simulink subsystem "PvtSubSys_PLAN_ALC"  (R2020b)
settings: Solver=VariableStepAuto  StartTime=0.0  StopTime=10.0  RelTol=1e-3
undefined symbols (not defined in the file or in its folder): P_Global_WheelBase_m, P_Global_WheelTrack_m, P_PLAN_ALC_DPCConfirmTimeHMI, P_PLAN_ALC_DPCExtraMultiFrameConfirmCntDrv, P_PLAN_ALC_DPCExtraMultiFrameConfirmCntNoh, P_PLAN_ALC_DPCExtraMultiFrameConfirmCntOverTk, P_PLAN_ALC_DPCthresholdLcDrvLv1, P_PLAN_ALC_DPCthresholdLcDrvLv2, P_PLAN_ALC_DPCthresholdLcDrvLv3, P_PLAN_ALC_DynamicDPCthreshold, P_PLAN_ALC_FWheelPreTime, P_PLAN_ALC_LcCancelDPCThreshold, P_PLAN_ALC_LcCancelLaneChangeReqDspTimeCnt, P_PLAN_ALC_LcCancelRoadWidthOffset, P_PLAN_ALC_LcCancelRoadWidthOffsetForDPC, P_PLAN_ALC_LcCurvatureInhibitionValueBrkPoints, P_PLAN_ALC_LcCurvatureInhibitionValueTable, P_PLAN_ALC_LcDelayCntSetNoh, P_PLAN_ALC_LcDelayCntSetOverTk, P_PLAN_ALC_LCDeltaTmeGap, P_PLAN_ALC_LcDrv_DyDiffThreshold, P_PLAN_ALC_LcDrvHMILineValidFtime, P_PLAN_ALC_LcEnterLane_factor, P_PLAN_ALC_LcFinishDyDiffBrkPoint, P_PLAN_ALC_LcFinishDyDiffRwFactorForAP, P_PLAN_ALC_LcFinishDyDiffRwFactorForHMI, P_PLAN_ALC_LcFinishDyDiffTableValue, P_PLAN_ALC_LciDrvExistDefaultDisp, P_PLAN_ALC_LciOverTkDeltaSpdLv1, P_PLAN_ALC_LciOverTkDeltaSpdLv2, P_PLAN_ALC_LciOverTkDeltaSpdLv3, P_PLAN_ALC_LcOverTkDPCthreshold, P_PLAN_ALC_LcOverTkRearVehTTClimit, P_PLAN_ALC_NOHLcSwt, P_PLAN_ALC_NOHTurnSts, P_PLAN_ALC_OverTkCutOutDyRWFactor, P_PLAN_ALC_OveTkrSupDist, P_PLAN_ALC_PreCurvatureFactor, P_PLAN_ALC_PreCurvaturePreTime, P_PLAN_ALC_TurnLmpType, P_PLAN_ALC_vMinPreLC_Drv, P_PLAN_ALC_vMinPreLC_Noh, P_PLAN_ALC_vMinPreLC_OverTk, P_PLAN_LcCancelTestEnable, PLAN_ALC_DangerObjIndex, PLAN_ALC_LcCancelReason, PLAN_ALC_LcDecsLe, PLAN_ALC_LcDecsRi, PLAN_ALC_LcFeReason, PLAN_ALC_LcReason, PLAN_ALC_sts, PLAN_ALC_stsReason, PLAN_ALC_TurnLightReq
libraries: simulink x198, TrueDurationTime x21, RisingEdgeTimer x2, JumpDetectionUint x1
(part 4 of 4)

== system PvtSubSys_PLAN_ALC/PLAN_IPHMI/Subsystem1 ==
  note: 0x1:need to lanechange but Conds not Satisfied
      | 0x2: ready to lanechange
  note: 该信号表示存在换道指示但不满足部分条件
  In1 : Inport
  LineValid : Inport  Port=2
  DPC : Inport  Port=3
  DPC_OnComing : Inport  Port=4
  LciDrvRi : Inport  Port=5
  AND : Logic  Commented=on  Inputs=4  AllPortsSameDT=off  OutDataTypeStr=boolean
  AND1 : Logic  Commented=on  AllPortsSameDT=off  OutDataTypeStr=boolean
  AND4 : Logic  AllPortsSameDT=off  OutDataTypeStr=boolean
  Bus Selector1 : BusSelector  Commented=on  OutputSignals=PLAN_ALC_LcDrvLe_IPVehSpd,PLAN_ALC_LcDrvLe_NoOnComing,PLAN_ALC_LcDrvLe_DPC,PLAN_ALC_LcDrvLe_LineValid,PLAN_ALC_LcDrvLe_LciDrv
  Chart1 : Stateflow chart  Commented=on  TreatAsAtomicUnit=on
  Chart2 : Stateflow chart  Commented=on  TreatAsAtomicUnit=on
  Compare To Constant : simulink/Logic and Bit Operations/Compare To Constant  Commented=on  relop=<=  const=P_PLAN_ALC_LcDrvHMILineValidFtime  OutDataTypeStr=boolean
  Compare To Constant1 : simulink/Logic and Bit Operations/Compare To Constant  relop=>  const=P_PLAN_ALC_LcDrvHMILineValidFtime  OutDataTypeStr=boolean
  Compare To Constant2 : simulink/Logic and Bit Operations/Compare To Constant  relop=>  const=P_PLAN_ALC_DynamicDPCthreshold  OutDataTypeStr=boolean
  Compare To Constant3 : simulink/Logic and Bit Operations/Compare To Constant  Commented=on  relop=<  const=P_PLAN_ALC_DynamicDPCthreshold  OutDataTypeStr=boolean
  Compare To Constant4 : simulink/Logic and Bit Operations/Compare To Constant  Commented=on  relop=>  const=P_PLAN_ALC_DPCConfirmTimeHMI  OutDataTypeStr=boolean
  Compare To Constant5 : simulink/Logic and Bit Operations/Compare To Constant  relop=>  const=P_PLAN_ALC_LcDrvHMILineValidFtime  OutDataTypeStr=boolean
  Constant7 : Constant  OutDataTypeStr=uint8
  Constant8 : Constant  Value=P_PLAN_ALC_LciDrvExistDefaultDisp  OutDataTypeStr=uint8
  Constant9 : Constant  Value=0  OutDataTypeStr=uint8
  NOT : Logic  Commented=on  Operator=NOT  IconShape=distinctive  AllPortsSameDT=off  OutDataTypeStr=boolean
  NOT1 : Logic  Operator=NOT  IconShape=distinctive  AllPortsSameDT=off  OutDataTypeStr=boolean
  NOT2 : Logic  Operator=NOT  IconShape=distinctive  AllPortsSameDT=off  OutDataTypeStr=boolean
  OR : Logic  Commented=on  Operator=OR  AllPortsSameDT=off  OutDataTypeStr=boolean
  OR1 : Logic  Commented=on  Operator=OR  AllPortsSameDT=off  OutDataTypeStr=boolean
  OR2 : Logic  Operator=OR  Inputs=4  AllPortsSameDT=off  OutDataTypeStr=boolean
  OR4 : Logic  AllPortsSameDT=off  OutDataTypeStr=boolean
  Switch : Switch  Criteria=u2 ~= 0
  Switch1 : Switch  Criteria=u2 ~= 0
  Terminator : Terminator  Commented=on
  TrueDurationTime1 : TrueDurationTime/TrueDurationTime  TCycle=0.02
  TrueDurationTime2 : TrueDurationTime/TrueDurationTime  Commented=on  TCycle=0.02
  TrueDurationTime3 : TrueDurationTime/TrueDurationTime  Commented=on  TCycle=0.02
  TrueDurationTime4 : TrueDurationTime/TrueDurationTime  TCycle=0.02
  LcDrvSatisfiedStsRi : Outport
  wires:
  Compare To Constant5/1 -> OR2/3
  TrueDurationTime4/1 -> Compare To Constant5/1
  NOT1/1 -> TrueDurationTime4/1
  In1/1 -> NOT1/1
  TrueDurationTime2/1 -> Compare To Constant4/1
  Compare To Constant3/1 -> TrueDurationTime2/1
  Chart2/1(LcSts) -> Terminator/1
  OR/1 -> AND/3
  OR1/1 -> AND/4
  NOT/1 -> AND1/2, TrueDurationTime3/1
  TrueDurationTime3/1 -> Compare To Constant/1
  AND1/1 -> OR/2, OR1/2
  AND/1 -> Chart2/1(LcConds)
  Compare To Constant/1 -> AND1/1
  DPC_OnComing/1 -> OR2/4
  Constant9/1 -> Switch1/3
  Bus Selector1/3 -> OR/1  "<PLAN_ALC_LcDrvLe_DPC>"
  AND4/1 -> Switch/2
  Bus Selector1/4 -> NOT/1, OR1/1  "<PLAN_ALC_LcDrvLe_LineValid>"
  Constant8/1 -> Switch1/1
  OR2/1 -> AND4/1  "LcNotSatisfied"
  Switch1/1 -> Switch/3
  NOT2/1 -> TrueDurationTime1/1
  TrueDurationTime1/1 -> Compare To Constant1/1
  Compare To Constant1/1 -> OR2/2
  Bus Selector1/1 -> AND/1  "<PLAN_ALC_LcDrvLe_IPVehSpd>"
  Constant7/1 -> Switch/1
  Bus Selector1/2 -> AND/2  "<PLAN_ALC_LcDrvLe_NoOnComing>"
  Compare To Constant2/1 -> OR4/1
  LineValid/1 -> OR4/2, NOT2/1
  Switch/1 -> LcDrvSatisfiedStsRi/1  "LcDrvSatisfiedStsRi"
  LciDrvRi/1 -> Switch1/2, AND4/2
  Bus Selector1/5 -> Chart2/2(LcReq)  "<PLAN_ALC_LcDrvLe_LciDrv>"
  DPC/1 -> Compare To Constant2/1
  Compare To Constant4/1 -> Chart1/1(on)
  OR4/1 -> OR2/1

== system PvtSubSys_PLAN_ALC/PLAN_IPHMI/Subsystem2 ==
  note: 0x1:need to lanechange but Conds not Satisfied
      | 0x2: ready to lanechange
  note: 该信号表示存在换道指示但不满足部分条件
  LineValid : Inport
  DPC : Inport  Port=2
  LciDrvLe : Inport  Port=3
  AND : Logic  Commented=on  Inputs=4  AllPortsSameDT=off  OutDataTypeStr=boolean
  AND1 : Logic  Commented=on  AllPortsSameDT=off  OutDataTypeStr=boolean
  AND4 : Logic  AllPortsSameDT=off  OutDataTypeStr=boolean
  Bus Selector1 : BusSelector  Commented=on  OutputSignals=PLAN_ALC_LcDrvLe_IPVehSpd,PLAN_ALC_LcDrvLe_NoOnComing,PLAN_ALC_LcDrvLe_DPC,PLAN_ALC_LcDrvLe_LineValid,PLAN_ALC_LcDrvLe_LciDrv
  Chart1 : Stateflow chart  Commented=on  TreatAsAtomicUnit=on
  Chart2 : Stateflow chart  Commented=on  TreatAsAtomicUnit=on
  Compare To Constant : simulink/Logic and Bit Operations/Compare To Constant  Commented=on  relop=<=  const=P_PLAN_ALC_LcDrvHMILineValidFtime  OutDataTypeStr=boolean
  Compare To Constant2 : simulink/Logic and Bit Operations/Compare To Constant  relop=>  const=P_PLAN_ALC_DynamicDPCthreshold  OutDataTypeStr=boolean
  Compare To Constant3 : simulink/Logic and Bit Operations/Compare To Constant  Commented=on  relop=<  const=P_PLAN_ALC_DynamicDPCthreshold  OutDataTypeStr=boolean
  Compare To Constant4 : simulink/Logic and Bit Operations/Compare To Constant  Commented=on  relop=>  const=P_PLAN_ALC_DPCConfirmTimeHMI  OutDataTypeStr=boolean
  Constant7 : Constant  OutDataTypeStr=uint8
  Constant8 : Constant  Value=P_PLAN_ALC_LciDrvExistDefaultDisp  OutDataTypeStr=uint8
  Constant9 : Constant  Value=0  OutDataTypeStr=uint8
  NOT : Logic  Commented=on  Operator=NOT  IconShape=distinctive  AllPortsSameDT=off  OutDataTypeStr=boolean
  OR : Logic  Commented=on  Operator=OR  AllPortsSameDT=off  OutDataTypeStr=boolean
  OR1 : Logic  Commented=on  Operator=OR  AllPortsSameDT=off  OutDataTypeStr=boolean
  OR4 : Logic  AllPortsSameDT=off  OutDataTypeStr=boolean
  Switch : Switch  Criteria=u2 ~= 0
  Switch1 : Switch  Criteria=u2 ~= 0
  Terminator : Terminator  Commented=on
  TrueDurationTime2 : TrueDurationTime/TrueDurationTime  Commented=on  TCycle=0.02
  TrueDurationTime3 : TrueDurationTime/TrueDurationTime  Commented=on  TCycle=0.02
  LcNohSatisfiedStsLe : Outport
  wires:
  TrueDurationTime2/1 -> Compare To Constant4/1
  Compare To Constant3/1 -> TrueDurationTime2/1
  Chart2/1(LcSts) -> Terminator/1
  OR/1 -> AND/3
  OR1/1 -> AND/4
  NOT/1 -> AND1/2, TrueDurationTime3/1
  TrueDurationTime3/1 -> Compare To Constant/1
  AND1/1 -> OR/2, OR1/2
  AND/1 -> Chart2/1(LcConds)
  Compare To Constant/1 -> AND1/1
  Constant9/1 -> Switch1/3
  Bus Selector1/3 -> OR/1  "<PLAN_ALC_LcDrvLe_DPC>"
  AND4/1 -> Switch/2
  Bus Selector1/4 -> NOT/1, OR1/1  "<PLAN_ALC_LcDrvLe_LineValid>"
  Constant8/1 -> Switch1/1
  OR4/1 -> AND4/1  "LcNotSatisfied"
  Switch1/1 -> Switch/3
  Bus Selector1/1 -> AND/1  "<PLAN_ALC_LcDrvLe_IPVehSpd>"
  Constant7/1 -> Switch/1
  Bus Selector1/2 -> AND/2  "<PLAN_ALC_LcDrvLe_NoOnComing>"
  Compare To Constant2/1 -> OR4/1
  LineValid/1 -> OR4/2
  Switch/1 -> LcNohSatisfiedStsLe/1  "LcNohSatisfiedStsLe"
  LciDrvLe/1 -> Switch1/2, AND4/2
  Bus Selector1/5 -> Chart2/2(LcReq)  "<PLAN_ALC_LcDrvLe_LciDrv>"
  DPC/1 -> Compare To Constant2/1
  Compare To Constant4/1 -> Chart1/1(on)

== system PvtSubSys_PLAN_ALC/PLAN_IPHMI/Subsystem3 ==
  note: 0x1:need to lanechange but Conds not Satisfied
      | 0x2: ready to lanechange
  note: 该信号表示存在换道指示但不满足部分条件
  LineValid : Inport
  DPC : Inport  Port=2
  LciDrvRi : Inport  Port=3
  AND : Logic  Commented=on  Inputs=4  AllPortsSameDT=off  OutDataTypeStr=boolean
  AND1 : Logic  Commented=on  AllPortsSameDT=off  OutDataTypeStr=boolean
  AND4 : Logic  AllPortsSameDT=off  OutDataTypeStr=boolean
  Bus Selector1 : BusSelector  Commented=on  OutputSignals=PLAN_ALC_LcDrvLe_IPVehSpd,PLAN_ALC_LcDrvLe_NoOnComing,PLAN_ALC_LcDrvLe_DPC,PLAN_ALC_LcDrvLe_LineValid,PLAN_ALC_LcDrvLe_LciDrv
  Chart1 : Stateflow chart  Commented=on  TreatAsAtomicUnit=on
  Chart2 : Stateflow chart  Commented=on  TreatAsAtomicUnit=on
  Compare To Constant : simulink/Logic and Bit Operations/Compare To Constant  Commented=on  relop=<=  const=P_PLAN_ALC_LcDrvHMILineValidFtime  OutDataTypeStr=boolean
  Compare To Constant2 : simulink/Logic and Bit Operations/Compare To Constant  relop=>  const=P_PLAN_ALC_DynamicDPCthreshold  OutDataTypeStr=boolean
  Compare To Constant3 : simulink/Logic and Bit Operations/Compare To Constant  Commented=on  relop=<  const=P_PLAN_ALC_DynamicDPCthreshold  OutDataTypeStr=boolean
  Compare To Constant4 : simulink/Logic and Bit Operations/Compare To Constant  Commented=on  relop=>  const=P_PLAN_ALC_DPCConfirmTimeHMI  OutDataTypeStr=boolean
  Constant7 : Constant  OutDataTypeStr=uint8
  Constant8 : Constant  Value=P_PLAN_ALC_LciDrvExistDefaultDisp  OutDataTypeStr=uint8
  Constant9 : Constant  Value=0  OutDataTypeStr=uint8
  NOT : Logic  Commented=on  Operator=NOT  IconShape=distinctive  AllPortsSameDT=off  OutDataTypeStr=boolean
  OR : Logic  Commented=on  Operator=OR  AllPortsSameDT=off  OutDataTypeStr=boolean
  OR1 : Logic  Commented=on  Operator=OR  AllPortsSameDT=off  OutDataTypeStr=boolean
  OR4 : Logic  AllPortsSameDT=off  OutDataTypeStr=boolean
  Switch : Switch  Criteria=u2 ~= 0
  Switch1 : Switch  Criteria=u2 ~= 0
  Terminator : Terminator  Commented=on
  TrueDurationTime2 : TrueDurationTime/TrueDurationTime  Commented=on  TCycle=0.02
  TrueDurationTime3 : TrueDurationTime/TrueDurationTime  Commented=on  TCycle=0.02
  LcNohSatisfiedStsRi : Outport
  wires:
  TrueDurationTime2/1 -> Compare To Constant4/1
  Compare To Constant3/1 -> TrueDurationTime2/1
  Chart2/1(LcSts) -> Terminator/1
  OR/1 -> AND/3
  OR1/1 -> AND/4
  NOT/1 -> AND1/2, TrueDurationTime3/1
  TrueDurationTime3/1 -> Compare To Constant/1
  AND1/1 -> OR/2, OR1/2
  AND/1 -> Chart2/1(LcConds)
  Compare To Constant/1 -> AND1/1
  Constant9/1 -> Switch1/3
  Bus Selector1/3 -> OR/1  "<PLAN_ALC_LcDrvLe_DPC>"
  AND4/1 -> Switch/2
  Bus Selector1/4 -> NOT/1, OR1/1  "<PLAN_ALC_LcDrvLe_LineValid>"
  Constant8/1 -> Switch1/1
  OR4/1 -> AND4/1  "LcNotSatisfied"
  Switch1/1 -> Switch/3
  Bus Selector1/1 -> AND/1  "<PLAN_ALC_LcDrvLe_IPVehSpd>"
  Constant7/1 -> Switch/1
  Bus Selector1/2 -> AND/2  "<PLAN_ALC_LcDrvLe_NoOnComing>"
  Compare To Constant2/1 -> OR4/1
  LineValid/1 -> OR4/2
  Switch/1 -> LcNohSatisfiedStsRi/1  "LcNohSatisfiedStsRi"
  LciDrvRi/1 -> Switch1/2, AND4/2
  Bus Selector1/5 -> Chart2/2(LcReq)  "<PLAN_ALC_LcDrvLe_LciDrv>"
  DPC/1 -> Compare To Constant2/1
  Compare To Constant4/1 -> Chart1/1(on)

== system PvtSubSys_PLAN_ALC/PLAN_IPHMI/Subsystem4 ==
  note: 该信号表示存在换道指示但不满足部分条件
  note: 0x1:need to lanechange but Conds not Satisfied
      | 0x2: ready to lanechange
  LineValid : Inport
  DPC : Inport  Port=2
  LciDrvRi : Inport  Port=3
  AND : Logic  Commented=on  Inputs=4  AllPortsSameDT=off  OutDataTypeStr=boolean
  AND1 : Logic  Commented=on  AllPortsSameDT=off  OutDataTypeStr=boolean
  AND4 : Logic  AllPortsSameDT=off  OutDataTypeStr=boolean
  Bus Selector1 : BusSelector  Commented=on  OutputSignals=PLAN_ALC_LcDrvLe_IPVehSpd,PLAN_ALC_LcDrvLe_NoOnComing,PLAN_ALC_LcDrvLe_DPC,PLAN_ALC_LcDrvLe_LineValid,PLAN_ALC_LcDrvLe_LciDrv
  Chart1 : Stateflow chart  Commented=on  TreatAsAtomicUnit=on
  Chart2 : Stateflow chart  Commented=on  TreatAsAtomicUnit=on
  Compare To Constant : simulink/Logic and Bit Operations/Compare To Constant  Commented=on  relop=<=  const=P_PLAN_ALC_LcDrvHMILineValidFtime  OutDataTypeStr=boolean
  Compare To Constant1 : simulink/Logic and Bit Operations/Compare To Constant  relop=>  const=P_PLAN_ALC_LcDrvHMILineValidFtime  OutDataTypeStr=boolean
  Compare To Constant2 : simulink/Logic and Bit Operations/Compare To Constant  relop=>  const=P_PLAN_ALC_DynamicDPCthreshold  OutDataTypeStr=boolean
  Compare To Constant3 : simulink/Logic and Bit Operations/Compare To Constant  Commented=on  relop=<  const=P_PLAN_ALC_DynamicDPCthreshold  OutDataTypeStr=boolean
  Compare To Constant4 : simulink/Logic and Bit Operations/Compare To Constant  Commented=on  relop=>  const=P_PLAN_ALC_DPCConfirmTimeHMI  OutDataTypeStr=boolean
  Constant7 : Constant  OutDataTypeStr=uint8
  Constant8 : Constant  Value=P_PLAN_ALC_LciDrvExistDefaultDisp  OutDataTypeStr=uint8
  Constant9 : Constant  Value=0  OutDataTypeStr=uint8
  Ground : Ground
  NOT : Logic  Commented=on  Operator=NOT  IconShape=distinctive  AllPortsSameDT=off  OutDataTypeStr=boolean
  NOT2 : Logic  Operator=NOT  IconShape=distinctive  AllPortsSameDT=off  OutDataTypeStr=boolean
  OR : Logic  Commented=on  Operator=OR  AllPortsSameDT=off  OutDataTypeStr=boolean
  OR1 : Logic  Commented=on  Operator=OR  AllPortsSameDT=off  OutDataTypeStr=boolean
  OR2 : Logic  Operator=OR  Inputs=3  AllPortsSameDT=off  OutDataTypeStr=boolean
  OR4 : Logic  AllPortsSameDT=off  OutDataTypeStr=boolean
  Switch : Switch  Criteria=u2 ~= 0
  Switch1 : Switch  Criteria=u2 ~= 0
  Terminator : Terminator  Commented=on
  TrueDurationTime1 : TrueDurationTime/TrueDurationTime  TCycle=0.02
  TrueDurationTime2 : TrueDurationTime/TrueDurationTime  Commented=on  TCycle=0.02
  TrueDurationTime3 : TrueDurationTime/TrueDurationTime  Commented=on  TCycle=0.02
  LcMrcSatisfiedStsRi : Outport
  wires:
  OR4/1 -> OR2/1
  Compare To Constant4/1 -> Chart1/1(on)
  DPC/1 -> Compare To Constant2/1
  Bus Selector1/5 -> Chart2/2(LcReq)  "<PLAN_ALC_LcDrvLe_LciDrv>"
  LciDrvRi/1 -> AND4/2, Switch1/2
  Switch/1 -> LcMrcSatisfiedStsRi/1  "LcNohSatisfiedStsRi"
  LineValid/1 -> NOT2/1, OR4/2
  Compare To Constant2/1 -> OR4/1
  Bus Selector1/2 -> AND/2  "<PLAN_ALC_LcDrvLe_NoOnComing>"
  Constant7/1 -> Switch/1
  Bus Selector1/1 -> AND/1  "<PLAN_ALC_LcDrvLe_IPVehSpd>"
  Compare To Constant1/1 -> OR2/2
  TrueDurationTime1/1 -> Compare To Constant1/1
  NOT2/1 -> TrueDurationTime1/1
  Switch1/1 -> Switch/3
  OR2/1 -> AND4/1  "LcNotSatisfied"
  Constant8/1 -> Switch1/1
  Bus Selector1/4 -> OR1/1, NOT/1  "<PLAN_ALC_LcDrvLe_LineValid>"
  AND4/1 -> Switch/2
  Bus Selector1/3 -> OR/1  "<PLAN_ALC_LcDrvLe_DPC>"
  Constant9/1 -> Switch1/3
  Compare To Constant/1 -> AND1/1
  AND/1 -> Chart2/1(LcConds)
  AND1/1 -> OR1/2, OR/2
  TrueDurationTime3/1 -> Compare To Constant/1
  NOT/1 -> TrueDurationTime3/1, AND1/2
  OR1/1 -> AND/4
  OR/1 -> AND/3
  Chart2/1(LcSts) -> Terminator/1
  Compare To Constant3/1 -> TrueDurationTime2/1
  TrueDurationTime2/1 -> Compare To Constant4/1
  Ground/1 -> OR2/3

== system PvtSubSys_PLAN_ALC/LcCancelFinishCalc1/Subsystem3/LPF ==
  signal : Inport
  Constant1 : Constant  Value=0.1
  MATLAB Function2 : MATLAB Function  TreatAsAtomicUnit=on
  Unit Delay2 : UnitDelay  SampleTime=-1  HasFrameUpgradeWarning=on
  result : Outport
  wires:
  MATLAB Function2/1(result) -> result/1, Unit Delay2/1
  Unit Delay2/1 -> MATLAB Function2/3(resultK1)
  Constant1/1 -> MATLAB Function2/1(Alpha)
  signal/1 -> MATLAB Function2/2(signal)

== system PvtSubSys_PLAN_ALC/LcCancelFinishCalc1/Subsystem3/Simulink Function ==
  note: 预测车体上的点或者固连在车体上的点的位置
  f : TriggerPort  TriggerType=function-call  IsSimulinkFunction=on  FunctionName=PointPre  FunctionVisibility=scoped  VariantControl=(inherit)
  Bus Selector : BusSelector  OutputSignals=mPrePointX,mPrePointY
  Bus Creator : BusCreator  Inputs=2
  Bus Creator1 : BusCreator  Inputs=2
  If : If  IfExpression=u1 == 0
  Merge : Merge
  Subsystem : Subsystem
  Subsystem1 : Subsystem
  u : ArgIn  DisableCoverage=on  OutDataTypeStr=single  ArgumentName=mPointX
  u1 : ArgIn  DisableCoverage=on  Port=2  OutDataTypeStr=single  ArgumentName=mPointY
  u2 : ArgIn  DisableCoverage=on  Port=3  OutDataTypeStr=single  ArgumentName=kapTraj
  u3 : ArgIn  DisableCoverage=on  Port=4  OutDataTypeStr=single  ArgumentName=mpsTrajSpd
  u4 : ArgIn  DisableCoverage=on  Port=5  OutDataTypeStr=single  ArgumentName=sPreTime
  y : ArgOut  DisableCoverage=on  OutDataTypeStr=single  ArgumentName=mPrePointX
  y1 : ArgOut  DisableCoverage=on  Port=2  OutDataTypeStr=single  ArgumentName=mPrePointY
  wires:
  Subsystem/1(mPrePointX) -> Bus Creator/1
  If/1 -> Subsystem1/Action
  Subsystem1/2(mPrePointY) -> Bus Creator1/2
  Subsystem1/1(mPrePointX) -> Bus Creator1/1
  u3/1 -> Subsystem1/1(mpsTrajSpd), Subsystem/2(mpsTrajSpd)
  Bus Creator/1 -> Merge/1
  Bus Selector/2 -> y1/1  "<mPrePointY>"
  Subsystem/2(mPrePointY) -> Bus Creator/2
  Merge/1 -> Bus Selector/1
  u/1 -> Subsystem1/3(mPointX), Subsystem/4(mPointX)
  u2/1 -> If/1, Subsystem/1(kapTraj)
  If/2 -> Subsystem/Action
  u4/1 -> Subsystem1/2(sPreTime), Subsystem/3(sPreTime)
  u1/1 -> Subsystem1/4(mPointY), Subsystem/5(mPointY)
  Bus Selector/1 -> y/1  "<mPrePointX>"
  Bus Creator1/1 -> Merge/2

== system PvtSubSys_PLAN_ALC/LcCancelFinishCalc1/Subsystem3/Simulink Function1 ==
  FrenetCS : TriggerPort  TriggerType=function-call  IsSimulinkFunction=on  FunctionName=FrenetCS  FunctionVisibility=scoped  VariantControl=(inherit)
  Add : Sum  Inputs=+++
  Add1 : Sum
  Add2 : Sum
  Constant : Constant  OutDataTypeStr=Inherit: Inherit via back propagation
  Divide : Product  Inputs=*/
  Gain : Gain  Gain=2
  Math Function : Math  Operator=square  SaturateOnIntegerOverflow=on
  Math Function1 : Math  Operator=square  SaturateOnIntegerOverflow=on
  Product : Product
  Product1 : Product
  Product2 : Product
  Sqrt : Sqrt  SaturateOnIntegerOverflow=on
  Subtract1 : Sum  Inputs=+-
  u : ArgIn  DisableCoverage=on  OutDataTypeStr=single  ArgumentName=LaneC0
  u1 : ArgIn  DisableCoverage=on  Port=2  OutDataTypeStr=single  ArgumentName=LaneC1
  u2 : ArgIn  DisableCoverage=on  Port=3  OutDataTypeStr=single  ArgumentName=LaneC2
  u4 : ArgIn  DisableCoverage=on  Port=4  OutDataTypeStr=single  ArgumentName=PointX
  u5 : ArgIn  DisableCoverage=on  Port=5  OutDataTypeStr=single  ArgumentName=PointY
  y1 : ArgOut  DisableCoverage=on  OutDataTypeStr=single  ArgumentName=PointFrenetD
  wires:
  u1/1 -> Add1/1, Product/2
  u4/1 -> Product/1, Math Function/1, Product2/2
  u2/1 -> Product1/2, Product2/1
  Math Function/1 -> Product1/1
  Product/1 -> Add/1
  Product1/1 -> Add/2
  u/1 -> Add/3
  Product2/1 -> Gain/1
  Gain/1 -> Add1/2
  Add1/1 -> Math Function1/1
  Math Function1/1 -> Add2/1
  Constant/1 -> Add2/2
  Add2/1 -> Sqrt/1
  Add/1 -> Subtract1/2
  Sqrt/1 -> Divide/2
  u5/1 -> Subtract1/1
  Divide/1 -> y1/1
  Subtract1/1 -> Divide/1

== system PvtSubSys_PLAN_ALC/LcOverTk/Subsystem5/Counter1 ==
  Trigger : Inport
  Constant3 : Constant  OutDataTypeStr=uint16
  Constant4 : Constant  Value=0  OutDataTypeStr=uint16
  Saturation1 : Saturate  UpperLimit=65000  LowerLimit=0
  Sum : Sum  Inputs=++|
  Switch : Switch  Criteria=u2 ~= 0
  Switch1 : Switch  Criteria=u2 ~= 0
  Unit Delay : UnitDelay  SampleTime=-1  HasFrameUpgradeWarning=on
  Cnt : Outport
  wires:
  Constant4/1 -> Switch/3, Switch1/3
  Constant3/1 -> Switch/1
  Switch1/1 -> Saturation1/1
  Switch/1 -> Sum/2
  Unit Delay/1 -> Sum/1
  Trigger/1 -> Switch/2, Switch1/2
  Sum/1 -> Switch1/1
  Saturation1/1 -> Cnt/1, Unit Delay/1

== system PvtSubSys_PLAN_ALC/LcOverTk/Subsystem5/Counter2 ==
  Trigger : Inport
  Constant3 : Constant  OutDataTypeStr=uint16
  Constant4 : Constant  Value=0  OutDataTypeStr=uint16
  Saturation1 : Saturate  UpperLimit=65000  LowerLimit=0
  Sum : Sum  Inputs=++|
  Switch : Switch  Criteria=u2 ~= 0
  Switch1 : Switch  Criteria=u2 ~= 0
  Unit Delay : UnitDelay  SampleTime=-1  HasFrameUpgradeWarning=on
  Cnt : Outport
  wires:
  Saturation1/1 -> Unit Delay/1, Cnt/1
  Sum/1 -> Switch1/1
  Trigger/1 -> Switch1/2, Switch/2
  Unit Delay/1 -> Sum/1
  Switch/1 -> Sum/2
  Switch1/1 -> Saturation1/1
  Constant3/1 -> Switch/1
  Constant4/1 -> Switch1/3, Switch/3

== system PvtSubSys_PLAN_ALC/LcOverTk/Subsystem5/Counter3 ==
  Trigger : Inport
  Constant3 : Constant  OutDataTypeStr=uint16
  Constant4 : Constant  Value=0  OutDataTypeStr=uint16
  Saturation1 : Saturate  UpperLimit=65000  LowerLimit=0
  Sum : Sum  Inputs=++|
  Switch : Switch  Criteria=u2 ~= 0
  Switch1 : Switch  Criteria=u2 ~= 0
  Unit Delay : UnitDelay  SampleTime=-1  HasFrameUpgradeWarning=on
  Cnt : Outport
  wires:
  Saturation1/1 -> Unit Delay/1, Cnt/1
  Sum/1 -> Switch1/1
  Trigger/1 -> Switch1/2, Switch/2
  Unit Delay/1 -> Sum/1
  Switch/1 -> Sum/2
  Switch1/1 -> Saturation1/1
  Constant3/1 -> Switch/1
  Constant4/1 -> Switch1/3, Switch/3

== system PvtSubSys_PLAN_ALC/LcOverTk/Subsystem5/Counter4 ==
  Trigger : Inport
  Constant3 : Constant  OutDataTypeStr=uint16
  Constant4 : Constant  Value=0  OutDataTypeStr=uint16
  Saturation1 : Saturate  UpperLimit=65000  LowerLimit=0
  Sum : Sum  Inputs=++|
  Switch : Switch  Criteria=u2 ~= 0
  Switch1 : Switch  Criteria=u2 ~= 0
  Unit Delay : UnitDelay  SampleTime=-1  HasFrameUpgradeWarning=on
  Cnt : Outport
  wires:
  Saturation1/1 -> Unit Delay/1, Cnt/1
  Sum/1 -> Switch1/1
  Trigger/1 -> Switch1/2, Switch/2
  Unit Delay/1 -> Sum/1
  Switch/1 -> Sum/2
  Switch1/1 -> Saturation1/1
  Constant3/1 -> Switch/1
  Constant4/1 -> Switch1/3, Switch/3

== system PvtSubSys_PLAN_ALC/LcOverTk/Subsystem5/Counter5 ==
  Trigger : Inport
  Constant3 : Constant  OutDataTypeStr=uint16
  Constant4 : Constant  Value=0  OutDataTypeStr=uint16
  Saturation1 : Saturate  UpperLimit=65000  LowerLimit=0
  Sum : Sum  Inputs=++|
  Switch : Switch  Criteria=u2 ~= 0
  Switch1 : Switch  Criteria=u2 ~= 0
  Unit Delay : UnitDelay  SampleTime=-1  HasFrameUpgradeWarning=on
  Cnt : Outport
  wires:
  Saturation1/1 -> Unit Delay/1, Cnt/1
  Sum/1 -> Switch1/1
  Trigger/1 -> Switch1/2, Switch/2
  Unit Delay/1 -> Sum/1
  Switch/1 -> Sum/2
  Switch1/1 -> Saturation1/1
  Constant3/1 -> Switch/1
  Constant4/1 -> Switch1/3, Switch/3

== system PvtSubSys_PLAN_ALC/LcCancelFinishCalc1/Subsystem3/Simulink Function/Subsystem ==
  kapTraj : Inport
  mpsTrajSpd : Inport  Port=2
  sPreTime : Inport  Port=3
  mPointX : Inport  Port=4
  mPointY : Inport  Port=5
  Action Port : ActionPort
  Add2 : Sum  Inputs=++-
  Add3 : Sum  Inputs=+++
  Cos : Trigonometry  Operator=cos
  Math Function : Math  Operator=reciprocal  SaturateOnIntegerOverflow=on
  Product : Product  Inputs=3
  Product{1,4,7..10} (6 alike) : Product
  Sin : Trigonometry
  Subtract : Sum  Inputs=+-
  mPrePointX : Outport
  mPrePointY : Outport  Port=2
  wires:
  Add2/1 -> mPrePointX/1  "mPrePointX"
  Add3/1 -> mPrePointY/1  "mPrePointY"
  mPointY/1 -> Product8/1, Product10/1
  Product4/1 -> Add2/2
  mPointX/1 -> Product9/1, Product4/1
  Product8/1 -> Add2/3
  Cos/1 -> Product7/2, Product4/2, Product10/2
  Product10/1 -> Add3/3
  Product9/1 -> Add3/2
  Sin/1 -> Product1/2, Product8/2, Product9/2
  Subtract/1 -> Add3/1  "PreVehDy"
  Product1/1 -> Add2/1  "PreVehDx"
  mpsTrajSpd/1 -> Product/2
  sPreTime/1 -> Product/3
  Product7/1 -> Subtract/2
  Product/1 -> Cos/1, Sin/1  "preAngle"
  Math Function/1 -> Subtract/1, Product7/1, Product1/1  "radius"
  kapTraj/1 -> Product/1, Math Function/1

== system PvtSubSys_PLAN_ALC/LcCancelFinishCalc1/Subsystem3/Simulink Function/Subsystem1 ==
  mpsTrajSpd : Inport
  sPreTime : Inport  Port=2
  mPointX : Inport  Port=3
  mPointY : Inport  Port=4
  Action Port : ActionPort
  Add2 : Sum
  Product : Product
  mPrePointX : Outport
  mPrePointY : Outport  Port=2
  wires:
  mpsTrajSpd/1 -> Product/1
  sPreTime/1 -> Product/2
  mPointY/1 -> mPrePointY/1  "mPrePointY"
  mPointX/1 -> Add2/2
  Add2/1 -> mPrePointX/1  "mPrePointX"
  Product/1 -> Add2/1  "PreVehDx"

== stateflow chart PvtSubSys_PLAN_ALC/LcCancelFinishCalc1/Chart ==
  state LeLc
    state LeLc1
      en:
      LaneInvalidCancelEnable=true;
      ex:
      LaneInvalidCancelEnable=false;
    state LeLc2
      en:
      LeLcFinishValid=true;
      ex:
      LeLcFinishValid=false;
    (default) -> LeLc1
    LeLc1 -> LeLc2 : [LeLaneCross]
  state CC
    LeLcFinishValid=false;
    RiLcFinishValid=false;
    LaneInvalidCancelEnable=false;
  state RiLc
    state RiLc1
      en:
      LaneInvalidCancelEnable=true;
      ex:
      LaneInvalidCancelEnable=false;
    state RiLc2
      en:
      RiLcFinishValid=true;
      ex:
      RiLcFinishValid=false;
    (default) -> RiLc1
    RiLc1 -> RiLc2 : [RiLaneCross]
  (default) -> CC
  CC -> LeLc [order 1] : [ALC_sts==2]
  CC -> RiLc [order 2] : [ALC_sts==3]
  RiLc -> CC : [ALC_sts~=3]
  LeLc -> CC : [ALC_sts~=2]
  data: LeLaneCross input; RiLaneCross input; ALC_sts input; LeLcFinishValid output; RiLcFinishValid output; LaneInvalidCancelEnable output

== matlab function PvtSubSys_PLAN_ALC/LcCancelFinishCalc1/Subsystem3/LPF/MATLAB Function2 ==
  data: Alpha input; signal input; result output; resultK1 input single
function result  = LowPassFilter(Alpha,signal,resultK1)
    result = Alpha*(signal - resultK1) + resultK1;
end

== stateflow chart PvtSubSys_PLAN_ALC/ALC_DECS ==
  state ALC_ON
    state LeLC
      en:
      LcCntLe=uint16(0);
      du:
      if LcDelayCnt > uint8(0)
      LcDelayCnt=LcDelayCnt-uint8(1);
      end
      if LcDelayCnt == uint8(0) && LcCntLe < uint16(65000)
      LcCntLe=LcCntLe+uint16(1);
      end
      if LcCntLe > uint16(0)
      ALC_Sts = uint8(2);
      end
      ex:
      LcCntLe = uint16(0);
      LcDelayCnt = uint8(0)
    state WaitLC%WaitLC
      en:
      ALC_Sts=uint8(1);%巡航
      ALC_LampReq=uint8(0);
      du:
      if LcFinishCntLe > 0
      LcFinishCntLe=LcFinishCntLe - uint8(1);
      end
      if LcCancelCntLe > 0
      LcCancelCntLe=LcCancelCntLe-uint8(1);
      end
      if LcFinishCntRi > 0
      LcFinishCntRi=LcFinishCntRi-uint8(1);
      end
      if LcCancelCntRi > 0
      LcCancelCntRi=LcCancelCntRi-uint8(1);
      end
      if(LcFinishCntLe==uint8(0) && LcCancelCntLe==uint8(0) && LcFinishCntRi==uint8(0) && LcCancelCntRi==uint8(0))
      LcReason=uint8(0);
      end
      ex:
      LcFinishCntLe=uint8(0);
      LcFinishCntRi=uint8(0);
      LcCancelCntLe=uint8(0);
      LcCancelCntRi=uint8(0);
    state RiLC
      en:
      LcCntRi=uint16(0);
      du:
      if LcDelayCnt > uint8(0)
      LcDelayCnt=LcDelayCnt-uint8(1);
      end
      if LcDelayCnt == uint8(0) && LcCntRi < uint16(65000)
      LcCntRi=LcCntRi+uint16(1);
      end
      if LcCntRi > uint16(0)
      ALC_Sts = uint8(3);
      end
      ex:
      LcCntRi=uint16(0);
      LcDelayCnt = uint8(0);
    WaitLC%WaitLC -> LeLC [order 1] : [LcfeLeDrv]
        | {LcReason=uint8(1);}
    WaitLC%WaitLC -> LeLC [order 3] : [LcfeLePilot]
        | {LcReason=uint8(2);
        | ALC_LampReq=uint8(1);
        | LcDelayCnt=LcDelayCntSetNoh;}
    WaitLC%WaitLC -> LeLC [order 5] : [LcfeLeOverTk]
        | {LcReason=uint8(4);
        | ALC_LampReq=uint8(1);
        | LcDelayCnt=LcDelayCntSetOverTk;}
    LeLC -> WaitLC%WaitLC [order 1] : [LcFinishLe && LcCntLe > 10]
        | {LcFinishCntLe = uint8(150);}
    LeLC -> WaitLC%WaitLC [order 2] : [LcCancelLe || LcCntLe > 1000]
        | {LcCancelCntLe = uint8(150);}
    (default) -> WaitLC%WaitLC
    WaitLC%WaitLC -> RiLC [order 7] : [LcMrcRi]
        | {LcReason=uint8(8);
        | ALC_LampReq=uint8(2);
        | LcDelayCnt=uint8(50);
        | LcFinishCntRi = uint8(150);}
    WaitLC%WaitLC -> RiLC [order 2] : [LcfeRiDrv]
        | {LcReason=uint8(1);}
    WaitLC%WaitLC -> RiLC [order 4] : [LcfeRiPilot]
        | {LcReason=uint8(2);
        | ALC_LampReq=uint8(2);
        | LcDelayCnt=LcDelayCntSetNoh;}
    WaitLC%WaitLC -> RiLC [order 6] : [LcfeRiOverTk]
        | {LcReason=uint8(4);
        | ALC_LampReq=uint8(2);
        | LcDelayCnt=LcDelayCntSetOverTk;}
    RiLC -> WaitLC%WaitLC [order 1] : [LcFinishRi && LcCntRi > 10]
        | {LcFinishCntRi = uint8(150);}
    RiLC -> WaitLC%WaitLC [order 2] : [LcCancelRi || LcCntRi > 1000]
        | {LcCancelCntRi = uint8(150);}
  state ALC_OFF
    ALC_Sts=uint8(0);%不可换道
    LcFinishCntLe=uint8(0);
    LcFinishCntRi=uint8(0);
    LcReason=uint8(0);
    LcCntLe=uint16(0);
    LcCntRi=uint16(0);
    ALC_LampReq=uint8(0);
    LcDelayCnt=uint8(0);
    ex:
    LcFinishCntRi=uint8(0);
    LcFinishCntLe=uint8(0);
  ALC_OFF -> ALC_ON : [ActiveALC]
  ALC_ON -> ALC_OFF : [~ActiveALC]
  (default) -> ALC_OFF
  data: ActiveALC input boolean size=1; LcMrcRi input; LcfeLeDrv input boolean size=1; LcfeRiDrv input boolean size=1; LcfeLePilot input; LcfeRiPilot input; LcfeLeOverTk input; LcfeRiOverTk input; ALC_Sts output uint8 size=1; ALC_LampReq output; LcCancelLe input boolean size=1; LcCancelRi input boolean size=1; LcFinishLe input boolean size=1; LcFinishRi input; LcReason output; LcCounter local; LcFinishCntLe output; LcFinishCntRi output; LcCancelCntLe output; LcCancelCntRi output; LcCntLe output; LcCntRi output; LcDelayCntSetNoh input; LcDelayCntSetOverTk input; LcDelayCnt output

== stateflow chart PvtSubSys_PLAN_ALC/LC2APadapter/ALCHMISM ==
  state CC
    LcAccSts=uint8(0);
    LcCnt=uint16(0);
  state Lc
    LcAccSts=uint8(1);
    en:
    LcCnt=uint16(0);
    du:
    LcCnt=min(LcCnt+uint16(1),uint16(2000));
  (default) -> CC
  CC -> Lc : [Lc]
  Lc -> CC : [(CC&&LcCnt>10)...
      | ||LcCnt>1000]
  data: Lc input; CC input; LcAccSts output; LcCnt local

== stateflow chart PvtSubSys_PLAN_ALC/LC2APadapter/Chart ==
  note: Do not put any code along
      | the transitions that run
      | down the right side!
  (default) -> (junction 18)
  (junction 18) -> (junction 19) [order 1] : [ALC_sts == uint8(1) && LciLe && DPCLe >0.3]
  (junction 18) -> (junction 22) [order 2]
  (junction 19) -> (junction 20) : {NOH_Intention=int8(-1);}
  (junction 20) -> (junction 21)
  (junction 21) -> (junction 25)
  (junction 22) -> (junction 23) [order 1] : [ALC_sts == uint8(1) && LciRi && DPCRi >0.3]
  (junction 22) -> (junction 26) [order 2] : {NOH_Intention=int8(0);}
  (junction 23) -> (junction 24) : {NOH_Intention=int8(1);}
  (junction 24) -> (junction 25)
  (junction 25) -> (junction 27)
  (junction 27) -> (junction 26)
  (junction 26) -> (junction 28)
  data: ALC_sts input; LciLe input; LciRi input; NOH_Intention output; DPCLe input; DPCRi input

== stateflow chart PvtSubSys_PLAN_ALC/LCCANCELadapter1/SigValueHold1 ==
  state Hold
    en:
    Cnt=uint16(0);
    du:
    Cnt=min(Cnt+uint16(1),uint16(2000));
  state Through
    HoldValue= uint16(0);
  (default) -> Through
  Through -> Hold [order 1] : [Hold1]{HoldValue=Value1;}
  Through -> Hold [order 2] : [Hold2]{HoldValue=Value2;}
  Hold -> Through : [~Hold1&&~Hold2&&Cnt>uint16(100)]
  data: Hold1 input; Hold2 input; Value1 input; Value2 input; HoldValue output; Cnt local

== stateflow chart PvtSubSys_PLAN_ALC/LcDrv/SigValueHold1 ==
  state Hold
    en:
    HoldValue1=Value1;
    HoldValue2=Value2;
    HoldValue3=Value3;
    HoldValue4=Value4;
  state Through
    HoldValue1=Value1;
    HoldValue2=Value2;
    HoldValue3=Value3;
    HoldValue4=Value4;
  (default) -> Through
  Hold -> Through : [~Hold]
  Through -> Hold : [Hold]
  data: Hold input; Value1 input; Value2 input; Value3 input; HoldValue1 output; HoldValue2 output; HoldValue3 output; Value4 input; HoldValue4 output

== stateflow chart PvtSubSys_PLAN_ALC/LcDrv/SigValueHold3 ==
  state Hold
    en:
    HoldValue1=Value1;
    HoldValue2=Value2;
    HoldValue3=Value3;
    HoldValue4=Value4;
  state Through
    HoldValue1=Value1;
    HoldValue2=Value2;
    HoldValue3=Value3;
    HoldValue4=Value4;
  (default) -> Through
  Hold -> Through : [~Hold]
  Through -> Hold : [Hold]
  data: Hold input; Value1 input; Value2 input; Value3 input; HoldValue1 output; HoldValue2 output; HoldValue3 output; Value4 input; HoldValue4 output

== stateflow chart PvtSubSys_PLAN_ALC/LcOverTk/DrvCancelSup/Chart ==
  state off
    Sts=false;
    dis = single(0);
  state on
    Sts=true;
    du:
    dis = dis + (V_ego/single(3.6)) * 0.02;
  (default) -> off
  off -> on : [Trigger]
  on -> off : [Clear]
  data: Trigger input; V_ego input; Clear input; Sts output; dis output

== matlab function PvtSubSys_PLAN_ALC/LcOverTk/MATLAB Function ==
  data: C1 input; curvature output; C2 input; x input
function curvature = fcn(C1, C2 ,x)
curvature=2*abs(C2)/(1+(C1+2*C2*x)^2)^(3/2);
end

== matlab function PvtSubSys_PLAN_ALC/LcOverTk/Subsystem4/MATLAB Function ==
  data: Trigger input; TriggerK1 input; signal input; result output; resultK1 input single
function result  = LowPassFilter(Trigger,TriggerK1,signal,resultK1)
if  Trigger == true
    if TriggerK1 == true
        result = 0.025*(signal - resultK1) + resultK1;
    else
        result = signal;
    end
else
    result = signal;
end
end

== matlab function PvtSubSys_PLAN_ALC/LcOverTk/Subsystem4/SLPDyCalc ==
  data: ObjDx input; dDyDiffRelLine output; ObjDy input; LineValid input; LineC3 input; LineC2 input; LineC1 input; LineC0 input; LineRange input
function dDyDiffRelLine  = ...
    fcn(ObjDx, ObjDy,...
    LineValid, LineC3, LineC2,LineC1, LineC0, LineRange)
% #define
fInvalidValue = single(0);%无效值

%init
dDyDiffRelLine = fInvalidValue;
if LineValid
    %计算横向相对距离
    LineC3Factor = single(0);
    LineC2Factor = Interp4(0, 1, LineRange, 1, LineRange+20, 0.7, LineRange+40, 0, ObjDx);
    dLineObjDy=(LineC3Factor * LineC3 * ObjDx * ObjDx * ObjDx) + (LineC2Factor * LineC2 * ObjDx * ObjDx) + (LineC1 * ObjDx) + LineC0;
    dDyDiffRelLine = ObjDy-dLineObjDy; 
end
end
function Out = Interp4(x1,z1,x2,z2,x3,z3,x4,z4,In)  %线性插值
if In<=x1
    Out = single(z1);
elseif (In>x1)&&(In<=x2)
    Out = single(z1+ (In-x1)*(z2-z1)/(x2-x1));
elseif (In>x2)&&(In<=x3)
    Out = single(z2+ (In-x2)*(z3-z2)/(x3-x2));
elseif (In>x3)&&(In<=x4)
    Out = single(z3+ (In-x3)*(z4-z3)/(x4-x3));
else
    Out = single(z4);
end
end

== stateflow chart PvtSubSys_PLAN_ALC/LcOverTk/Subsystem5/SigHold1 ==
  state ture
    outData=Data;
    outTrigger=Trigger;
  state hold
    en:
    Cnt=uint8(0);
    du:
    if Cnt<uint8(255)
    Cnt=Cnt+uint8(1);
    end
  state cross
    outData=Data;
    outTrigger=Trigger;
  (default) -> ture
  cross -> ture : [Trigger]
  ture -> hold : [~Trigger]
  hold -> ture [order 1] : [Trigger]
  hold -> cross [order 2] : [Cnt>250]
  data: Data input; Trigger input; outData output; Cnt local; outTrigger output

== stateflow chart PvtSubSys_PLAN_ALC/LcOverTk/Subsystem5/SigHold2 ==
  state ture
    outData=Data;
    outTrigger=Trigger;
  state hold
    en:
    Cnt=uint8(0);
    du:
    if Cnt<uint8(255)
    Cnt=Cnt+uint8(1);
    end
  state cross
    outData=Data;
    outTrigger=Trigger;
  (default) -> ture
  cross -> ture : [Trigger]
  ture -> hold : [~Trigger]
  hold -> ture [order 1] : [Trigger]
  hold -> cross [order 2] : [Cnt>250]
  data: Data input; Trigger input; outData output; Cnt local; outTrigger output

== matlab function PvtSubSys_PLAN_ALC/LcOverTk/TurnReqCal2 ==
  data: LeftTurnReq output; SpdSetValue_kph input; P0ID input; P0Vr_ms input; VehicleSpd_kph input; tStartDecel input; NearestObjValid_L input; NearestObjValid_R input; NearestObjSpeed_L input; NearestObjSpeed_R input; DrivingOnTheMostLeftLane_b input; LCDeltaTmeGap input; RightTurnReq output; SpeedDeltaSetSpd_kph output; SpeedDelta_L_kph output; SpeedDelta_R_kph output; nPreLcInvalidID output uint8; LowSpdFlag output; DeltaSpd_kph input; nPreLcInvalidID_K1 input uint8; SpdSup input; SpdSuphappend_K1 input boolean; SpdSuphappend output boolean
function [LeftTurnReq,RightTurnReq, SpeedDeltaSetSpd_kph, SpeedDelta_L_kph,SpeedDelta_R_kph,nPreLcInvalidID,LowSpdFlag,SpdSuphappend]...
    = fcn(SpdSetValue_kph,P0ID,P0Vr_ms,VehicleSpd_kph,tStartDecel,...
    NearestObjValid_L,NearestObjValid_R,NearestObjSpeed_L,NearestObjSpeed_R,...
    DrivingOnTheMostLeftLane_b,LCDeltaTmeGap,...
    DeltaSpd_kph, nPreLcInvalidID_K1, SpdSup,SpdSuphappend_K1)

P0SpeedDisplay_kph = (((P0Vr_ms * 3.6) + VehicleSpd_kph) * 1.03) + 1.3;
SpeedDeltaSetSpd_kph = SpdSetValue_kph - P0SpeedDisplay_kph;
SpeedDeltaVehSpd_kph = SpdSetValue_kph - (VehicleSpd_kph * 1.03 + 1.3);
% TimeGap = P0Range / (max(VehicleSpd_kph,10) / 3.6);
P0VrG_ms = P0Vr_ms + (VehicleSpd_kph / 3.6);
SpeedDelta_L_kph = (NearestObjSpeed_L - P0VrG_ms) * 3.6;
SpeedDelta_R_kph = (NearestObjSpeed_R - P0VrG_ms) * 3.6;

nPreLcInvalidID=nPreLcInvalidID_K1;
SpdSuphappend=SpdSuphappend_K1;

LowSpdFlag=false;
bPreLcFlag=false; %压速换道-提前换道
bSupLcFlag=false;%压速换道-长时间被压速

%if P0ID==0x0 %如果P0丢失，则无效ID置0
    nPreLcInvalidID=0x0;
    SpdSuphappend=false;
%end

% if P0ID ~= 0x0 && abs(P0Vr_ms)<3 %如果P0实际车速已经差不多了，不对此目标触发压速换道的提前换道。
%     nPreLcInvalidID=P0ID;
% end

%换道时机处理
if (P0ID ~= 0x0)...
        && (SpeedDeltaSetSpd_kph >= DeltaSpd_kph)...%与P0速度差在15km/h以上
        && (tStartDecel <= LCDeltaTmeGap)...%提前换道触发时机
        && (P0ID ~= nPreLcInvalidID)
    bPreLcFlag=true;
end

% if (P0ID ~= 0x0)...   
%         && SpeedDeltaVehSpd_kph >= DeltaSpd_kph...
%         && (P0ID == nPreLcInvalidID)
%     LowSpdFlag=true;
% end

if SpdSup && ~SpdSuphappend
    bSupLcFlag=true;
    SpdSuphappend=true;
end


if bPreLcFlag || bSupLcFlag %评估左右目标
    if DrivingOnTheMostLeftLane_b==false && ((NearestObjValid_L == false) || ((NearestObjValid_L == true) && (SpeedDelta_L_kph > 15)))
        LeftTurnReq = true;
        RightTurnReq = false;
%         nPreLcInvalidID=P0ID; %已经触发过的P0，同一ID不再触发提前压速换道。
    elseif ((DrivingOnTheMostLeftLane_b == true) && ((NearestObjValid_R == false) || ((NearestObjValid_R == true) && (SpeedDelta_R_kph > 15)))) 
        LeftTurnReq = false;
        RightTurnReq = true;
%         nPreLcInvalidID=P0ID;
    else
        LeftTurnReq = false;
        RightTurnReq = false;
    end
else
    LeftTurnReq = false;
    RightTurnReq = false;
end

== stateflow chart PvtSubSys_PLAN_ALC/PLAN_IPHMI/ALCHMISM ==
  state CC
    HMILaneChanging=uint8(0);
    LcCnt=uint16(0);
  state Right
    HMILaneChanging=uint8(2);
    en:
    LcCnt=uint16(0);
    du:
    LcCnt=min(LcCnt+uint16(1),uint16(2000))
  state Left
    HMILaneChanging=uint8(1);
    en:
    LcCnt=uint16(0);
    du:
    LcCnt=min(LcCnt+uint16(1),uint16(2000));
  (default) -> CC
  CC -> Right [order 2] : [Right]
  CC -> Left [order 1] : [Left]
  Left -> CC : [(CC&&LcCnt>10)...
      | ||LcCnt>1000]
  Right -> CC : [(CC&&LcCnt>10)...
      | ||LcCnt>1000]
  data: Left input; Right input; CC input; HMILaneChanging output; LcCnt local

== stateflow chart PvtSubSys_PLAN_ALC/PLAN_IPHMI/Chart1 ==
  note: Input：
      | LcXXSatisfiedStsLe/Ri
      | 0x1: Req lanechange but Conds not Satisfied
      | 0x2: Ready to lanechange
  note: Output：
      | HWA_LaneChangeReq
      | 0x0:No display
      | 0x1:left satisfied
      | 0x2:right satisfied
      | 0x3:left not satisfied
      | 0x4:right not satisfied
  (default) -> (junction 92)
  (junction 92) -> (junction 98) [order 1] : [ HWAsts==uint8(3) && (LcDrvSatisfiedStsLe==uint8(1) || LcNohSatisfiedStsLe==uint8(1) || LcCancelLe) ]
  (junction 92) -> (junction 118) [order 2]
  (junction 98) -> (junction 94) : {HWA_LaneChangeReq=uint8(3);}
  (junction 94) -> (junction 121)
  (junction 121) -> (junction 123)
  (junction 118) -> (junction 114) [order 1] : [(HWAsts==uint8(3) && (LcDrvSatisfiedStsLe==uint8(2) || LcNohSatisfiedStsLe==uint8(2) || LcOverTkTurnLampReqLe )) || (HWAsts==uint8(5) && HMILaneChanging==uint8(1))]
  (junction 118) -> (junction 122) [order 2]
  (junction 114) -> (junction 119) : {HWA_LaneChangeReq=uint8(1);}
  (junction 119) -> (junction 123)
  (junction 123) -> (junction 96)
  (junction 122) -> (junction 104) [order 1] : [HWAsts==uint8(3) && (LcDrvSatisfiedStsRi==uint8(1) || LcNohSatisfiedStsRi==uint8(1) || LcMrcSatisfiedStsRi==uint8(1) || LcCancelRi) ]
  (junction 122) -> (junction 99) [order 2]
  (junction 104) -> (junction 85) : {HWA_LaneChangeReq=uint8(4);}
  (junction 85) -> (junction 96)
  (junction 96) -> (junction 97)
  (junction 99) -> (junction 111) [order 1] : [(HWAsts==uint8(3) && (LcDrvSatisfiedStsRi==uint8(2) || LcNohSatisfiedStsRi==uint8(2) || LcMrcSatisfiedStsRi == uint8(2) || LcOverTkTurnLampReqRi )) || (HWAsts==uint8(6) && HMILaneChanging==uint8(2))]
  (junction 99) -> (junction 101) [order 2] : {HWA_LaneChangeReq=uint8(0);}
  (junction 111) -> (junction 86) : {HWA_LaneChangeReq=uint8(2);}
  (junction 86) -> (junction 97)
  (junction 97) -> (junction 120)
  (junction 120) -> (junction 101)
  (junction 101) -> (junction 93)
  data: HMILaneChanging input; HWAsts input; LcDrvSatisfiedStsLe input; LcDrvSatisfiedStsRi input; LcNohSatisfiedStsLe input; LcNohSatisfiedStsRi input; LcMrcSatisfiedStsRi input; LcOverTkTurnLampReqLe input; LcOverTkTurnLampReqRi input; HWA_LaneChangeReq output; LcCancelLe input; LcCancelRi input

== stateflow chart PvtSubSys_PLAN_ALC/PLAN_IPHMI/Chart2 ==
  note: Input：
      | LcXXSatisfiedStsLe/Ri
      | 0x1: Req lanechange but Conds not Satisfied
      | 0x2: Ready to lanechange
  note: Output：
      | HWA_LaneChangeReq
      | 0x0:No display
      | 0x1:left satisfied
      | 0x2:right satisfied
      | 0x3:left not satisfied
      | 0x4:right not satisfied
  (default) -> (junction 92)
  (junction 92) -> (junction 98) [order 1] : [ HWAsts==uint8(3) && (LcDrvSatisfiedStsLe==uint8(1) || LcNohSatisfiedStsLe==uint8(1) || LcCancelLe) ]
  (junction 92) -> (junction 118) [order 2]
  (junction 98) -> (junction 94) : {HWA_LaneChangeReq=uint8(3);}
  (junction 94) -> (junction 121)
  (junction 121) -> (junction 123)
  (junction 118) -> (junction 114) [order 1] : [(HWAsts==uint8(3) && (LcDrvSatisfiedStsLe==uint8(2) || LcNohSatisfiedStsLe==uint8(2) || LcOverTkTurnLampReqLe )) || (HWAsts==uint8(5) && HMILaneChanging==uint8(1))]
  (junction 118) -> (junction 122) [order 2]
  (junction 114) -> (junction 119) : {HWA_LaneChangeReq=uint8(1);}
  (junction 119) -> (junction 123)
  (junction 123) -> (junction 96)
  (junction 122) -> (junction 104) [order 1] : [HWAsts==uint8(3) && (LcDrvSatisfiedStsRi==uint8(1) || LcNohSatisfiedStsRi==uint8(1) || LcCancelRi) ]
  (junction 122) -> (junction 99) [order 2]
  (junction 104) -> (junction 85) : {HWA_LaneChangeReq=uint8(4);}
  (junction 85) -> (junction 96)
  (junction 96) -> (junction 97)
  (junction 99) -> (junction 111) [order 1] : [(HWAsts==uint8(3) && (LcDrvSatisfiedStsRi==uint8(2) || LcNohSatisfiedStsRi==uint8(2) || LcOverTkTurnLampReqRi )) || (HWAsts==uint8(6) && HMILaneChanging==uint8(2))]
  (junction 99) -> (junction 101) [order 2] : {HWA_LaneChangeReq=uint8(0);}
  (junction 111) -> (junction 86) : {HWA_LaneChangeReq=uint8(2);}
  (junction 86) -> (junction 97)
  (junction 97) -> (junction 120)
  (junction 120) -> (junction 101)
  (junction 101) -> (junction 93)
  data: HMILaneChanging input; HWAsts input; LcDrvSatisfiedStsLe input; LcDrvSatisfiedStsRi input; LcNohSatisfiedStsLe input; LcNohSatisfiedStsRi input; LcOverTkTurnLampReqLe input; LcOverTkTurnLampReqRi input; HWA_LaneChangeReq output; LcCancelLe input; LcCancelRi input

== stateflow chart PvtSubSys_PLAN_ALC/PLAN_IPHMI/Subsystem/Chart1 ==
  state off
    out=false;
  state on
    out=true;
  (default) -> off
  on -> off : [off&&~on]
  off -> on : [on&&~off]
  data: on input; off input; out output

== stateflow chart PvtSubSys_PLAN_ALC/PLAN_IPHMI/Subsystem/Chart2 ==
  note: Do not put any code along
      | the transitions that run
      | down the right side!
  (default) -> (junction 64) : % 判断LCReq状态
  (junction 64) -> (junction 65) [order 1] : [ LcReq && LcConds]
  (junction 64) -> (junction 68) [order 2]
  (junction 65) -> (junction 66) : {LcSts=uint8(2);}
  (junction 66) -> (junction 67)
  (junction 67) -> (junction 71)
  (junction 68) -> (junction 69) [order 1] : [LcReq && ~LcConds]
  (junction 68) -> (junction 72) [order 2] : {LcSts=uint8(0);}
  (junction 69) -> (junction 70) : {LcSts=uint8(1);}
  (junction 70) -> (junction 71)
  (junction 71) -> (junction 75)
  (junction 75) -> (junction 72)
  (junction 72) -> (junction 82)
  data: LcConds input; LcReq input; LcSts output

== stateflow chart PvtSubSys_PLAN_ALC/PLAN_IPHMI/Subsystem1/Chart1 ==
  state off
    out=false;
  state on
    out=true;
  (default) -> off
  on -> off : [off&&~on]
  off -> on : [on&&~off]
  data: on input; off input; out output

== stateflow chart PvtSubSys_PLAN_ALC/PLAN_IPHMI/Subsystem1/Chart2 ==
  note: Do not put any code along
      | the transitions that run
      | down the right side!
  (default) -> (junction 64) : % 判断LCReq状态
  (junction 64) -> (junction 65) [order 1] : [ LcReq && LcConds]
  (junction 64) -> (junction 68) [order 2]
  (junction 65) -> (junction 66) : {LcSts=uint8(2);}
  (junction 66) -> (junction 67)
  (junction 67) -> (junction 71)
  (junction 68) -> (junction 69) [order 1] : [LcReq && ~LcConds]
  (junction 68) -> (junction 72) [order 2] : {LcSts=uint8(0);}
  (junction 69) -> (junction 70) : {LcSts=uint8(1);}
  (junction 70) -> (junction 71)
  (junction 71) -> (junction 75)
  (junction 75) -> (junction 72)
  (junction 72) -> (junction 82)
  data: LcConds input; LcReq input; LcSts output

== stateflow chart PvtSubSys_PLAN_ALC/PLAN_IPHMI/Subsystem2/Chart1 ==
  state off
    out=false;
  state on
    out=true;
  (default) -> off
  on -> off : [off&&~on]
  off -> on : [on&&~off]
  data: on input; off input; out output

== stateflow chart PvtSubSys_PLAN_ALC/PLAN_IPHMI/Subsystem2/Chart2 ==
  note: Do not put any code along
      | the transitions that run
      | down the right side!
  (default) -> (junction 64) : % 判断LCReq状态
  (junction 64) -> (junction 65) [order 1] : [ LcReq && LcConds]
  (junction 64) -> (junction 68) [order 2]
  (junction 65) -> (junction 66) : {LcSts=uint8(2);}
  (junction 66) -> (junction 67)
  (junction 67) -> (junction 71)
  (junction 68) -> (junction 69) [order 1] : [LcReq && ~LcConds]
  (junction 68) -> (junction 72) [order 2] : {LcSts=uint8(0);}
  (junction 69) -> (junction 70) : {LcSts=uint8(1);}
  (junction 70) -> (junction 71)
  (junction 71) -> (junction 75)
  (junction 75) -> (junction 72)
  (junction 72) -> (junction 82)
  data: LcConds input; LcReq input; LcSts output

== stateflow chart PvtSubSys_PLAN_ALC/PLAN_IPHMI/Subsystem3/Chart1 ==
  state off
    out=false;
  state on
    out=true;
  (default) -> off
  on -> off : [off&&~on]
  off -> on : [on&&~off]
  data: on input; off input; out output

== stateflow chart PvtSubSys_PLAN_ALC/PLAN_IPHMI/Subsystem3/Chart2 ==
  note: Do not put any code along
      | the transitions that run
      | down the right side!
  (default) -> (junction 64) : % 判断LCReq状态
  (junction 64) -> (junction 65) [order 1] : [ LcReq && LcConds]
  (junction 64) -> (junction 68) [order 2]
  (junction 65) -> (junction 66) : {LcSts=uint8(2);}
  (junction 66) -> (junction 67)
  (junction 67) -> (junction 71)
  (junction 68) -> (junction 69) [order 1] : [LcReq && ~LcConds]
  (junction 68) -> (junction 72) [order 2] : {LcSts=uint8(0);}
  (junction 69) -> (junction 70) : {LcSts=uint8(1);}
  (junction 70) -> (junction 71)
  (junction 71) -> (junction 75)
  (junction 75) -> (junction 72)
  (junction 72) -> (junction 82)
  data: LcConds input; LcReq input; LcSts output

== stateflow chart PvtSubSys_PLAN_ALC/PLAN_IPHMI/Subsystem4/Chart1 ==
  state off
    out=false;
  state on
    out=true;
  (default) -> off
  on -> off : [off&&~on]
  off -> on : [on&&~off]
  data: on input; off input; out output

== stateflow chart PvtSubSys_PLAN_ALC/PLAN_IPHMI/Subsystem4/Chart2 ==
  note: Do not put any code along
      | the transitions that run
      | down the right side!
  (default) -> (junction 64) : % 判断LCReq状态
  (junction 64) -> (junction 65) [order 1] : [ LcReq && LcConds]
  (junction 64) -> (junction 68) [order 2]
  (junction 65) -> (junction 66) : {LcSts=uint8(2);}
  (junction 66) -> (junction 67)
  (junction 67) -> (junction 71)
  (junction 68) -> (junction 69) [order 1] : [LcReq && ~LcConds]
  (junction 68) -> (junction 72) [order 2] : {LcSts=uint8(0);}
  (junction 69) -> (junction 70) : {LcSts=uint8(1);}
  (junction 70) -> (junction 71)
  (junction 71) -> (junction 75)
  (junction 75) -> (junction 72)
  (junction 72) -> (junction 82)
  data: LcConds input; LcReq input; LcSts output
